simulink model "HelicopterSimulation"  (R2017a)
settings: Solver=VariableStepAuto  StartTime=0.0  StopTime=10  RelTol=1e-3
libraries: simulink x1
settings Model: Creator=enzoevers  LastModifiedBy=enzoe

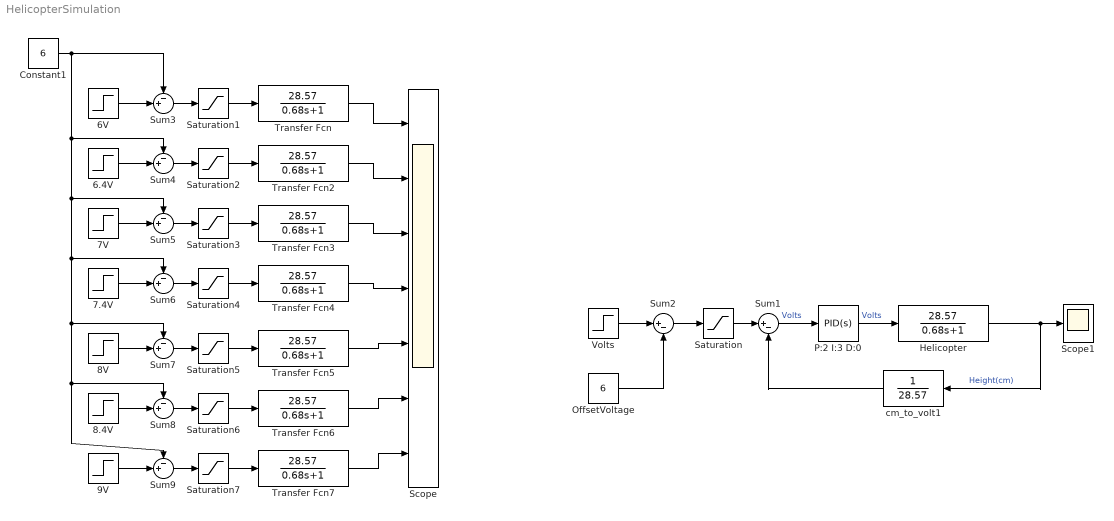
== system HelicopterSimulation ==
  6.4V : Step  Time=0  After=6.4  SampleTime=0
  6V : Step  Time=0  After=6  SampleTime=0
  7.4V : Step  Time=0  After=7.4  SampleTime=0
  7V : Step  Time=0  After=7  SampleTime=0
  8.4V : Step  Time=0  After=8.4  SampleTime=0
  "8V " : Step  Time=0  After=8  SampleTime=0
  9V : Step  Time=0  After=9  SampleTime=0
  Constant1 : Constant  Value=6
  Helicopter : TransferFcn  Numerator=[28.57]  Denominator=[0.68 1]
  "OffsetVoltage " : Constant  Value=6
  P:2 I:3 D:0 : simulink/Continuous/PID Controller  Controller=PID  TimeDomain=Continuous-time  SampleTime=-1  IntegratorMethod=Forward Euler  FilterMethod=Forward Euler  Form=Parallel  UseFilter=on  ControllerParametersSource=internal  P=2  I=3  D=0  N=100  InitialConditionSource=internal  InitialConditionForIntegrator=0  InitialConditionForFilter=0  ExternalReset=none  LimitOutput=off  UpperSaturationLimit=inf  LowerSaturationLimit=-inf  LinearizeAsGain=on  AntiWindupMode=none  Kb=1  TrackingMode=off  Kt=1  PParamMin=[]  PParamMax=[]  IParamMin=[]  IParamMax=[]  DParamMin=[]  DParamMax=[]  NParamMin=[]  NParamMax=[]  KbParamMin=[]  KbParamMax=[]  KtParamMin=[]  KtParamMax=[]  POutMin=[]  POutMax=[]  IOutMin=[]  IOutMax=[]  DOutMin=[]  DOutMax=[]  NOutMin=[]  NOutMax=[]  KbOutMin=[]  KbOutMax=[]  KtOutMin=[]  KtOutMax=[]  IntegratorOutMin=[]  IntegratorOutMax=[]  FilterOutMin=[]  FilterOutMax=[]  SumOutMin=[]  SumOutMax=[]  SumI1OutMin=[]  SumI1OutMax=[]  SumI2OutMin=[]  SumI2OutMax=[]  SumI3OutMin=[]  SumI3OutMax=[]  SumDOutMin=[]  SumDOutMax=[]  SaturationOutMin=[]  SaturationOutMax=[]  IntegratorContinuousStateAttributes=''  IntegratorStateMustResolveToSignalObject=off  IntegratorRTWStateStorageClass=Auto  FilterContinuousStateAttributes=''  FilterStateMustResolveToSignalObject=off  FilterRTWStateStorageClass=Auto  DifferentiatorICPrevScaledInput=0  DifferentiatorOutMin=[]  DifferentiatorOutMax=[]  InitialConditionSetting=State (most efficient)
  Saturation{,1..7} (8 alike) : Saturate  UpperLimit=10  LowerLimit=0
  Scope : Scope  NumInputPorts=7
  Scope1 : Scope
  Sum1 : Sum  Inputs=|+-
  Sum2 : Sum  Inputs=|+-
  Sum{3..9} (7 alike) : Sum  Inputs=-+|
  Transfer Fcn{,2..7} (7 alike) : TransferFcn  Numerator=[28.57]  Denominator=[0.68 1]
  Volts : Step  Time=0  After=7  SampleTime=0
  cm_to_volt1 : TransferFcn  Denominator=[0 28.57]
  wires:
  Transfer Fcn/1 -> Scope/1
  Saturation1/1 -> Transfer Fcn/1
  Helicopter/1 -> Scope1/1, cm_to_volt1/1  "Height(cm)"
  Sum1/1 -> P:2 I:3 D:0/1  "Volts"
  P:2 I:3 D:0/1 -> Helicopter/1  "Volts"
  Saturation/1 -> Sum1/1
  Sum3/1 -> Saturation1/1
  6V/1 -> Sum3/2
  Constant1/1 -> Sum9/1, Sum8/1, Sum7/1, Sum6/1, Sum5/1, Sum4/1, Sum3/1
  Transfer Fcn7/1 -> Scope/7
  Transfer Fcn6/1 -> Scope/6
  Transfer Fcn5/1 -> Scope/5
  Transfer Fcn4/1 -> Scope/4
  Transfer Fcn3/1 -> Scope/3
  Transfer Fcn2/1 -> Scope/2
  Saturation2/1 -> Transfer Fcn2/1
  Saturation3/1 -> Transfer Fcn3/1
  Saturation4/1 -> Transfer Fcn4/1
  Saturation5/1 -> Transfer Fcn5/1
  Saturation6/1 -> Transfer Fcn6/1
  Saturation7/1 -> Transfer Fcn7/1
  Sum4/1 -> Saturation2/1
  Sum5/1 -> Saturation3/1
  Sum6/1 -> Saturation4/1
  Sum7/1 -> Saturation5/1
  Sum8/1 -> Saturation6/1
  Sum9/1 -> Saturation7/1
  9V/1 -> Sum9/2
  8.4V/1 -> Sum8/2
  "8V "/1 -> Sum7/2
  7.4V/1 -> Sum6/2
  7V/1 -> Sum5/2
  6.4V/1 -> Sum4/2
  cm_to_volt1/1 -> Sum1/2
  Volts/1 -> Sum2/1
  "OffsetVoltage "/1 -> Sum2/2
  Sum2/1 -> Saturation/1
